simulink model "pulse_detector_v1"  (R2018b)
settings: Solver=VariableStepAuto  StartTime=0.0  StopTime=SimTime  RelTol=1e-3
undefined symbols (not defined in the file): CorrFilter, threshold, WindowLen
libraries: simulink x1, dspsrcs4 x1, hdlsllib x1
settings Model: Creator=cchung  LastModifiedBy=jerickso
settings DebuggingCC: LibraryContextMissingDiagnostic=none
settings SFSimCC: SimUseLocalCustomCode=off
settings RTWCC: RTWUseLocalCustomCode=off

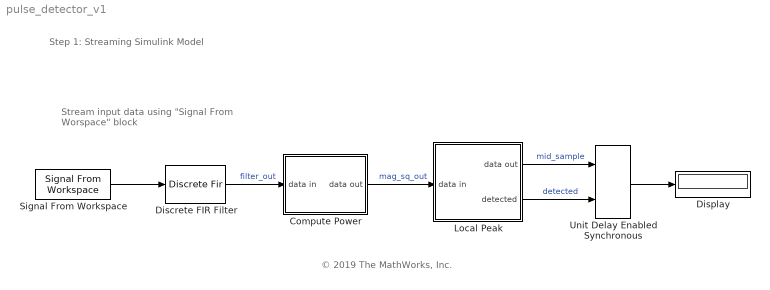
== system pulse_detector_v1 ==
  note: Step 1: Streaming Simulink Model
  note: Stream input data using
      | "Signal From Worspace" block
  note: © 2019 The MathWorks, Inc.
  Compute Power : Subsystem
  Discrete FIR Filter : DiscreteFir  Coefficients=CorrFilter
  Display : Display
  Local Peak : Subsystem
  Signal From Workspace : dspsrcs4/Signal From Workspace  X=RxSignal  Ts=1  nsamps=1  OutputAfterFinalValue=Setting to zero  ignoreOrWarnInputAndFrameLengths=off  OutputFrames=off
  Unit Delay Enabled Synchronous : hdlsllib/Discrete/Unit Delay Enabled Synchronous  InitialCondition=0.0  SampleTime=-1
      settings: SourceProductName=HDL Coder  SourceProductBaseCode=HD
  wires:
  Local Peak/2(detected) -> Unit Delay Enabled Synchronous/2  "detected"
  Compute Power/1(data out) -> Local Peak/1(data in)  "mag_sq_out"
  Discrete FIR Filter/1 -> Compute Power/1(data in)  "filter_out"
  Signal From Workspace/1 -> Discrete FIR Filter/1
  Local Peak/1(data out) -> Unit Delay Enabled Synchronous/1  "mid_sample"
  Unit Delay Enabled Synchronous/1 -> Display/1

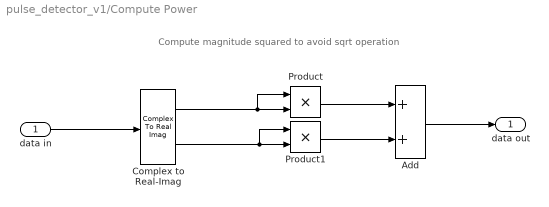
== system pulse_detector_v1/Compute Power ==
  note: Compute magnitude squared to avoid sqrt operation
  data in : Inport
  Add : Sum
  Complex to Real-Imag : ComplexToRealImag
  Product : Product
  Product1 : Product
  data out : Outport
  wires:
  Complex to Real-Imag/1 -> Product/1, Product/2
  Complex to Real-Imag/2 -> Product1/1, Product1/2
  Product1/1 -> Add/2
  Product/1 -> Add/1
  Add/1 -> data out/1
  data in/1 -> Complex to Real-Imag/1

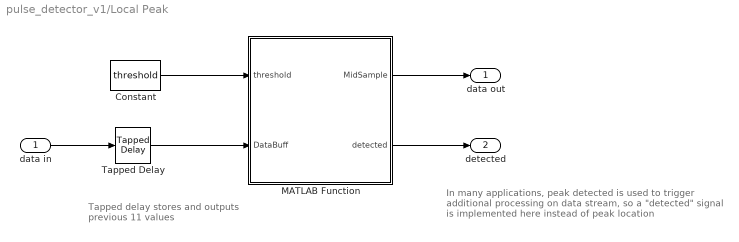
== system pulse_detector_v1/Local Peak ==
  note: Tapped delay stores and
      | outputs previous 11 values
  note: In many applications, peak detected is used
      | to trigger additional processing on data stream,
      | so a "detected" signal is implemented here
      | instead of peak location
  data in : Inport
  Constant : Constant  Value=threshold
  MATLAB Function : MATLAB Function  TreatAsAtomicUnit=on
  Tapped Delay : simulink/Discrete/Tapped Delay  vinit=0.0  samptime=-1  NumDelays=WindowLen  DelayOrder=Oldest  includeCurrent=off
  data out : Outport
  detected : Outport  Port=2
  wires:
  data in/1 -> Tapped Delay/1
  Tapped Delay/1 -> MATLAB Function/2(DataBuff)
  Constant/1 -> MATLAB Function/1(threshold)
  MATLAB Function/1(MidSample) -> data out/1
  MATLAB Function/2(detected) -> detected/1

== matlab function pulse_detector_v1/Local Peak/MATLAB Function ==
  data: WindowLen parameter; threshold input; DataBuff input; MidSample output; detected output
% Hardware friendly implementation of peak finder
%
% Function inputs:
% * WindowLen - non-tunable parameter defined under Simulink->Edit Data
% * threhold  - input port (connected to constant)
% * DataBuff  - input port (buffering done using Simulink block)
%
% Function outputs:
% * "detected" is set when MidSample is local max

function [MidSample,detected] = fcn(WindowLen, threshold, DataBuff)
%#codegen


MidIdx = ceil(WindowLen/2);

% Compare each value in the window to the middle sample via subtraction
MidSample = DataBuff(MidIdx);
CompareOut = DataBuff - MidSample; % this is a vector

% if all values in the result are negative and the middle sample is
% greater than a threshold, it is a local max
if all(CompareOut <= 0) && (MidSample > threshold)
    detected = 1;
else
    detected = 0;
end
